simulink model "vidu03"  (R2016a)
settings: Solver=VariableStepAuto  StartTime=0.0  StopTime=10000  RelTol=1e-3
settings Model: Creator=Lenovo  LastModifiedBy=Lenovo

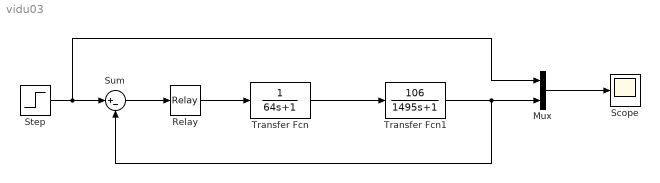
== system vidu03 ==
  Mux : Mux  Inputs=2
  Relay : Relay  OnSwitchValue=+2  OffSwitchValue=-2
  Scope : Scope
  Step : Step  Time=0  After=100  SampleTime=0
  Sum : Sum  Inputs=|+-
  Transfer Fcn : TransferFcn  Denominator=[64 1]
  Transfer Fcn1 : TransferFcn  Numerator=[106]  Denominator=[1495 1]
  wires:
  Mux/1 -> Scope/1
  Step/1 -> Mux/1, Sum/1
  Sum/1 -> Relay/1
  Relay/1 -> Transfer Fcn/1
  Transfer Fcn/1 -> Transfer Fcn1/1
  Transfer Fcn1/1 -> Mux/2, Sum/2
